simulink library "INT_Conv_GripIntrlck"  (R2016b)
settings: Solver=VariableStepAuto  StartTime=0.0  StopTime=10.0  RelTol=1e-3
settings Model: Creator=Administrator  LastModifiedBy=Administrator

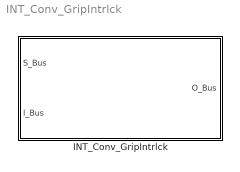
== system INT_Conv_GripIntrlck ==
  INT_Conv_GripIntrlck : Subsystem

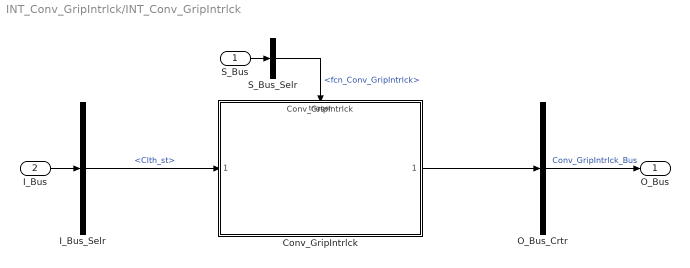
== system INT_Conv_GripIntrlck/INT_Conv_GripIntrlck ==
  S_Bus : Inport
  I_Bus : Inport  Port=2
  Conv_GripIntrlck : ModelReference  ModelNameDialog=Conv_GripIntrlck  SimulationMode=Normal  ModelReferenceVersion=1.2  TriggerPortName=function  TriggerPortTriggerType=function-call  TriggerPortStatesWhenEnabling=held
  I_Bus_Selr : BusSelector  OutputSignals=Clth_st
  O_Bus_Crtr : BusCreator  Inputs=1
  S_Bus_Selr : BusSelector  OutputSignals=fcn_Conv_GripIntrlck
  O_Bus : Outport
  wires:
  S_Bus_Selr/1 -> Conv_GripIntrlck/Trigger  "<fcn_Conv_GripIntrlck>"
  S_Bus/1 -> S_Bus_Selr/1
  I_Bus/1 -> I_Bus_Selr/1
  I_Bus_Selr/1 -> Conv_GripIntrlck/1  "<Clth_st>"
  O_Bus_Crtr/1 -> O_Bus/1  "Conv_GripIntrlck_Bus"
  Conv_GripIntrlck/1 -> O_Bus_Crtr/1
